simulink model "harmonic_comensation_simulation"  (R2020a)
settings: Solver=VariableStepAuto  StartTime=0.0  StopTime=3  RelTol=1e-3
values from neighbouring files (symbols this model uses):
  comp_table1 = [0.0466534535288 0.0494662824403 0.051313759182 0.0523377273586 0.0526570501043 0.0523721273536 0.0515686346954 0.0503206665416 0.0486934290661 0.0467455980054 0.0445314294364 0.0421026843564 ... (285300 elements, 951x300)]    [tables_50to1000.mat]
undefined symbols (not defined in the file or in its folder): B13, Bm, deltaT, DiscIntNeverNeededParam, J, Kd0, lam_pm, Ld, Lq, max_predq, P, Rs, run_comp, ss_d, ss_q, start_comp
libraries: simulink x1
settings Model: Creator=adamh  LastModifiedBy=adamh

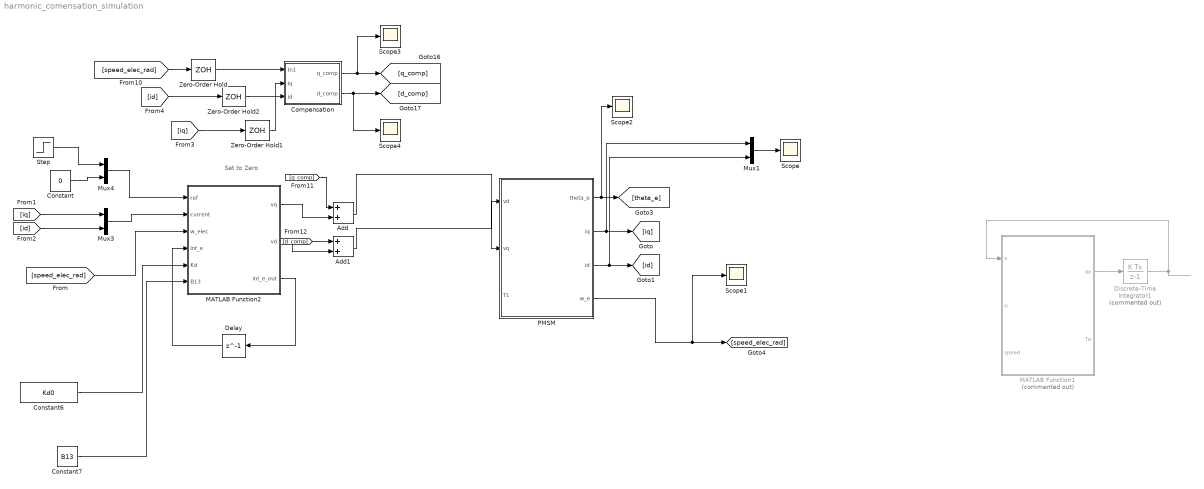
== system harmonic_comensation_simulation ==
  note: Set to Zero
  Add : Sum
  Add1 : Sum
  Compensation : Subsystem
  Constant : Constant  Value=0
  Constant6 : Constant  Value=Kd0
  Constant7 : Constant  Value=B13
  Delay : Delay  DelayLength=1  InitialCondition=[0.0; 0.0]
  Discrete-Time Integrator1 : DiscreteIntegrator  Commented=on  SampleTime=deltaT/100  ICPrevOutput=DiscIntNeverNeededParam  ICPrevScaledInput=DiscIntNeverNeededParam
  MATLAB Function1 : MATLAB Function  Commented=on  TreatAsAtomicUnit=on  SystemSampleTime=deltaT/100
  MATLAB Function2 : MATLAB Function  TreatAsAtomicUnit=on  SystemSampleTime=deltaT
  Mux1 : Mux  Inputs=2
  Mux3 : Mux  Inputs=2
  Mux4 : Mux  Inputs=2
  PMSM : Subsystem
  Scope{,1..4} (5 alike) : Scope
  Step : Step  Time=0  SampleTime=0
  Zero-Order Hold : ZeroOrderHold  SampleTime=deltaT
  Zero-Order Hold1 : ZeroOrderHold  SampleTime=deltaT
  Zero-Order Hold2 : ZeroOrderHold  SampleTime=deltaT
  wires:
  Constant6/1 -> MATLAB Function2/5(Kd)
  [d_comp] -> Add1/1
  Constant7/1 -> MATLAB Function2/6(B13)
  [q_comp] -> Add/1
  MATLAB Function2/2(vd) -> Add1/2
  Mux4/1 -> MATLAB Function2/1(ref)
  MATLAB Function2/1(vq) -> Add/2
  Delay/1 -> MATLAB Function2/4(int_e)
  Mux3/1 -> MATLAB Function2/2(current)
  [speed_elec_rad] -> MATLAB Function2/3(w_elec)
  Constant/1 -> Mux4/2
  [iq] -> Mux3/1
  [id] -> Mux3/2
  MATLAB Function2/3(int_e_out) -> Delay/1
  [speed_elec_rad] -> Zero-Order Hold/1
  Compensation/1(q_comp) -> Scope3/1, [q_comp]
  Compensation/2(d_comp) -> Scope4/1, [d_comp]
  Step/1 -> Mux4/1
  Zero-Order Hold/1 -> Compensation/1(In1)
  ? -> MATLAB Function1/2(u)
  Discrete-Time Integrator1/1 -> MATLAB Function1/1(x)
  MATLAB Function1/1(dx) -> Discrete-Time Integrator1/1
  Add/1 -> PMSM/2(vq)
  Add1/1 -> PMSM/1(vd)
  PMSM/4(w_e) -> Scope1/1, [speed_elec_rad]
  PMSM/1(theta_e) -> Scope2/1, [theta_e]
  PMSM/3(id) -> Mux1/2, [id]
  PMSM/2(iq) -> Mux1/1, [iq]
  Mux1/1 -> Scope/1
  [iq] -> Zero-Order Hold1/1
  [id] -> Zero-Order Hold2/1
  Zero-Order Hold1/1 -> Compensation/2(iq)
  Zero-Order Hold2/1 -> Compensation/3(id)

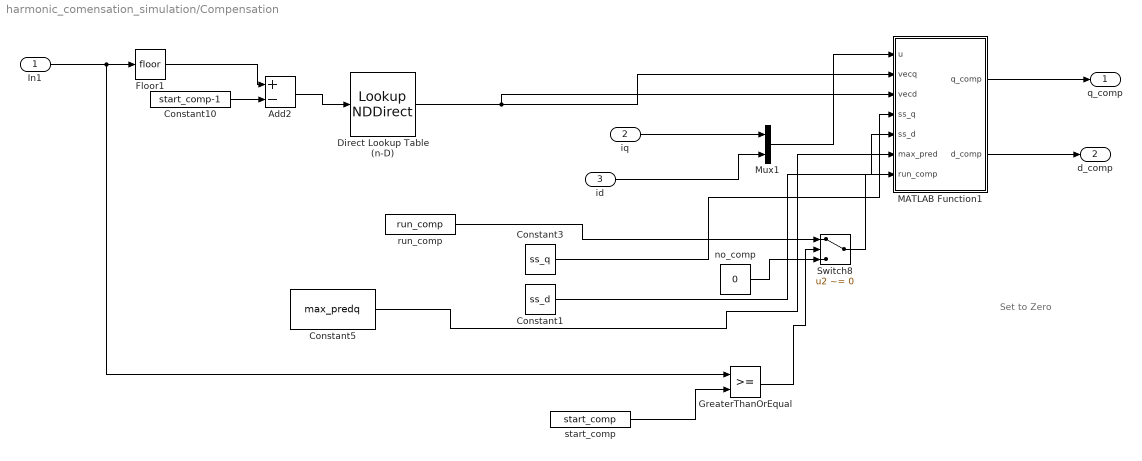
== system harmonic_comensation_simulation/Compensation ==
  note: Set to Zero
  In1 : Inport
  iq : Inport  Port=2
  id : Inport  Port=3
  Add2 : Sum  Inputs=+-
  Constant1 : Constant  Value=ss_d
  Constant10 : Constant  Value=start_comp-1
  Constant3 : Constant  Value=ss_q
  Constant5 : Constant  Value=max_predq
  Direct Lookup Table (n-D) : LookupNDDirect  InputsSelectThisObjectFromTable=Vector  Table=comp_table1'
  Floor1 : Rounding
  GreaterThanOrEqual : RelationalOperator  OutDataTypeStr=boolean  RndMeth=Simplest
  MATLAB Function1 : MATLAB Function  TreatAsAtomicUnit=on
  Mux1 : Mux  Inputs=2
  Switch8 : Switch  Criteria=u2 ~= 0
  no_comp : Constant  Value=0
  run_comp : Constant  Value=run_comp
  start_comp : Constant  Value=start_comp
  q_comp : Outport
  d_comp : Outport  Port=2
  wires:
  Add2/1 -> Direct Lookup Table (n-D)/1
  Direct Lookup Table (n-D)/1 -> MATLAB Function1/3(vecd), MATLAB Function1/2(vecq)
  GreaterThanOrEqual/1 -> Switch8/2
  id/1 -> Mux1/2
  run_comp/1 -> Switch8/1
  Mux1/1 -> MATLAB Function1/1(u)
  Constant10/1 -> Add2/2
  Floor1/1 -> Add2/1
  start_comp/1 -> GreaterThanOrEqual/2
  Constant5/1 -> MATLAB Function1/6(max_pred)
  Constant3/1 -> MATLAB Function1/4(ss_q)
  Constant1/1 -> MATLAB Function1/5(ss_d)
  no_comp/1 -> Switch8/3
  MATLAB Function1/2(d_comp) -> d_comp/1
  Switch8/1 -> MATLAB Function1/7(run_comp)
  MATLAB Function1/1(q_comp) -> q_comp/1
  In1/1 -> GreaterThanOrEqual/1, Floor1/1
  iq/1 -> Mux1/1

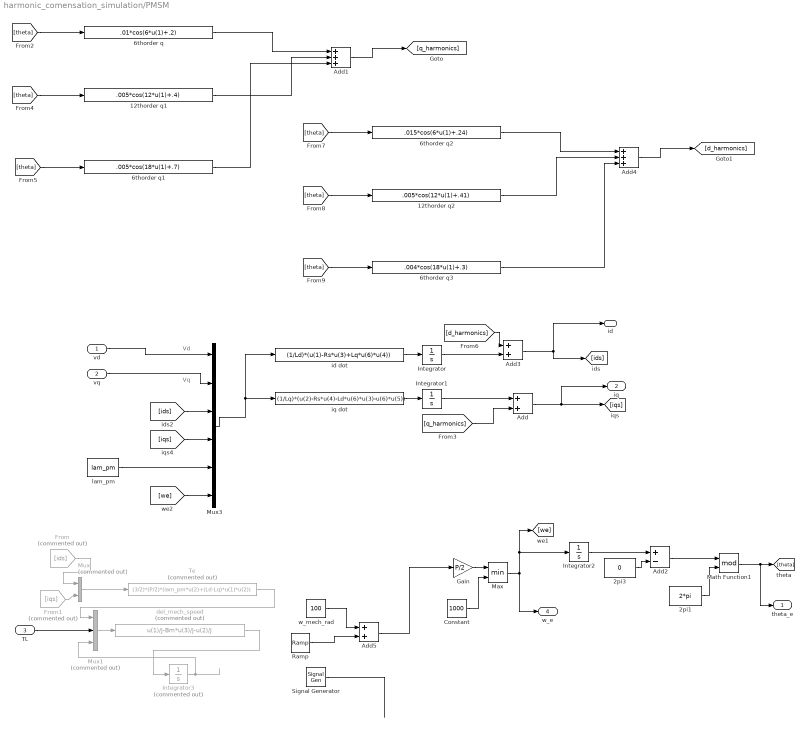
== system harmonic_comensation_simulation/PMSM ==
  note: Vq
  note: Vd
  vd : Inport
  vq : Inport  Port=2
  TL : Inport  Port=3
  12thorder q1 : Fcn  Expr=.005*cos(12*u(1)+.4)
  12thorder q2 : Fcn  Expr=.005*cos(12*u(1)+.41)
  2pi1 : Constant  Value=2*pi
  2pi3 : Constant  Value=0
  6thorder q : Fcn  Expr=.01*cos(6*u(1)+.2)
  6thorder q1 : Fcn  Expr=.005*cos(18*u(1)+.7)
  6thorder q2 : Fcn  Expr=.015*cos(6*u(1)+.24)
  6thorder q3 : Fcn  Expr=.004*cos(18*u(1)+.3)
  Add : Sum
  Add1 : Sum  Inputs=+++
  Add2 : Sum  Inputs=+-
  Add3 : Sum
  Add4 : Sum  Inputs=+++
  Add5 : Sum
  Constant : Constant  Value=1000
  From : From  Commented=on  GotoTag=ids
  From1 : From  Commented=on  GotoTag=iqs
  Gain : Gain  Gain=P/2
  Integrator : Integrator
  Integrator1 : Integrator
  Integrator2 : Integrator
  Integrator3 : Integrator  Commented=on
  Math Function1 : Math  Operator=mod  SignedPower=on  SaturateOnIntegerOverflow=on
  Max : MinMax  Inputs=2
  Mux : Mux  Commented=on  Inputs=2
  Mux1 : Mux  Commented=on  Inputs=3
  Mux3 : Mux  Inputs=6
  Ramp : simulink/Sources/Ramp  slope=25  start=1  InitialOutput=0
  Signal Generator : SignalGenerator  Amplitude=10  Units=rad/sec
  Te : Fcn  Commented=on  Expr=(3/2)*(P/2)*(lam_pm*u(2)+(Ld-Lq)*u(1)*u(2))
  del_mech_speed : Fcn  Commented=on  Expr=u(1)/J-Bm*u(3)/J-u(2)/J
  id dot : Fcn  Expr=(1/Ld)*(u(1)-Rs*u(3)+Lq*u(6)*u(4))
  iq dot : Fcn  Expr=(1/Lq)*(u(2)-Rs*u(4)-Ld*u(6)*u(3)-u(6)*u(5))
  lam_pm : Constant  Value=lam_pm
  w_mech_rad : Constant  Value=100
  theta_e : Outport  VectorParamsAs1DForOutWhenUnconnected=off
  iq : Outport  Port=2
  id : Outport  Port=3
  w_e : Outport  Port=4
  wires:
  Integrator/1 -> Add3/2
  iq dot/1 -> Integrator1/1
  id dot/1 -> Integrator/1
  vd/1 -> Mux3/1
  [iqs] -> Mux3/4
  Integrator2/1 -> Add2/1
  Mux3/1 -> iq dot/1, id dot/1
  [ids] -> Mux3/3
  lam_pm/1 -> Mux3/5
  [we] -> Mux3/6
  2pi1/1 -> Math Function1/2
  Math Function1/1 -> theta_e/1, [theta]
  2pi3/1 -> Add2/2
  Add2/1 -> Math Function1/1
  Integrator1/1 -> Add/1
  vq/1 -> Mux3/2
  Mux/1 -> Te/1
  From/1 -> Mux/1
  From1/1 -> Mux/2
  del_mech_speed/1 -> Integrator3/1
  Integrator3/1 -> Mux1/3
  Mux1/1 -> del_mech_speed/1
  Te/1 -> Mux1/1
  TL/1 -> Mux1/2
  6thorder q/1 -> Add1/1
  Add/1 -> iq/1, [iqs]
  [q_harmonics] -> Add/2
  12thorder q1/1 -> Add1/2
  6thorder q1/1 -> Add1/3
  Add1/1 -> [q_harmonics]
  [d_harmonics] -> Add3/1
  Add3/1 -> id/1, [ids]
  6thorder q3/1 -> Add4/3
  12thorder q2/1 -> Add4/2
  6thorder q2/1 -> Add4/1
  Add4/1 -> [d_harmonics]
  w_mech_rad/1 -> Add5/1
  Ramp/1 -> Add5/2
  Add5/1 -> Gain/1
  Gain/1 -> Max/1
  Constant/1 -> Max/2
  Max/1 -> Integrator2/1, [we], w_e/1
  Signal Generator/1 -> ?
  [theta] -> 6thorder q/1
  [theta] -> 6thorder q1/1
  [theta] -> 12thorder q1/1
  [theta] -> 6thorder q2/1
  [theta] -> 12thorder q2/1
  [theta] -> 6thorder q3/1

== matlab function harmonic_comensation_simulation/Compensation/MATLAB Function1 ==
  settings: updateMethod=DISCRETE
  data: u input; q_comp output; vecq input; vecd input; ss_q input; ss_d input; max_pred input; run_comp input; d_comp output
function [q_comp, d_comp]  = fcn(u,vecq,vecd, ss_q,ss_d, max_pred, run_comp)

    persistent delayq
    persistent q_pred
    persistent delayd
    persistent d_pred
    
    if isempty(delayq)  
        nEq = length(vecq);
        delayq = zeros(nEq,1);
    end
    if isempty(q_pred)  
        q_pred = 0;
    end
     if isempty(delayd)  
        nEd = length(vecd);
        delayd = zeros(nEd,1);
    end
    if isempty(d_pred)  
        d_pred = 0;
    end  

    
    % compensation
    %protection
    if abs(q_pred)>max_pred || run_comp == 0         
       delayq = [u(1);delayq(1:end-1)]; 
       q_pred = dot(vecq,delayq);
       q_comp=0;
    else

        delayq = [u(1)+q_pred;delayq(1:end-1)];
        q_pred = dot(vecq,delayq); % extract 
        q_comp = ss_q*q_pred;  
    end
    
    if abs(d_pred)>max_pred || run_comp == 0         
       delayd = [u(2);delayd(1:end-1)]; 
       d_pred = dot(vecd,delayd);
       d_comp=0;
    else
        delayd = [u(2)+d_pred;delayd(1:end-1)];
        d_pred = dot(vecd,delayd); % extract 
        d_comp = ss_d*d_pred; 
    end

== matlab function harmonic_comensation_simulation/MATLAB Function2 ==
  data: ref input size=2; current input size=2; w_elec input; int_e input size=2; vq output; vd output; int_e_out output; Kd input; B13 input
function [vq, vd, int_e_out] = traditional_LQI(ref,current,w_elec,int_e, Kd, B13)

% VDC = 42;

% from Real Parameters
% Ke =[1.6894   -0.1842    0.0000    0.3627   -1.7799    0.3569;
%     0.1842    1.6894   -0.3627    0.0000   -0.3569   -1.7799] ; 
% from fbedmdc
% Ke =[ 2.3940   -0.1699   -0.0016    0.5049   -2.5070    0.2027;
%     0.0938    2.4391   -0.5046   -0.0009   -0.1301   -2.5545];



e = ref - current;
int_e = int_e + e;
% int_e = int_e +Tsd2*e + Tsd2*old_e_in
Kd(1,2) = Kd(1,2)*w_elec;
% Ke(1,4) = Ke(1,4)*w_elec;
Kd(2,1) = Kd(2,1)*w_elec;
% Ke(2,3) = Ke(2,3)*w_elec;

% states = [u(1);u(2);u(1)*factor; u(2)*factor; int_e(1); int_e(2)];
states = [current(1);current(2); int_e(1); int_e(2)];

y = -Kd*states;
% y(1) = y(1) - B13*w_elec; % is B13 negative, should be
vq =y(1);
vd =y(2);

% vq = vq/VDC;
% vd =vd/VDC;

% vq = 0;
% vd = 0;


int_e_out = int_e;
% old_e = e;
% prevent integrator windup
% if vq ~= y(1) || vd ~= y(2)
%     %satureted
%     int_e_out = int_e - e;
% else
%     int_e_out = int_e;
% end

== matlab function harmonic_comensation_simulation/MATLAB Function1 ==
  data: x input size=4; u input size=2; dx output size=4; speed input; Te output; params parameter
function [dx, Te] = extended_pmsm_motor(x,u,speed, params)
    % extended dq model from Advanced Theory of Fractional-Slot
    % Concentrated Permanent Magnet Machines Thesis    

    % initial condition x(6) = .1631 Lq_dc    
    % initial condition x(7) = .1447 Ld_dc 
    % initial condition x(9) = .4055 Lamdapm_d
    
%     persistent dx_1_old dx_2_old  
%     if isempty(dx_1_old)
%         dx_1_old = 0;
%         dx_2_old = 0;
%     end
    
    vq = u(1);
    vd = u(2);

    rs = params.rs;
    Ld_dc = params.Ld_dc;
    Lq_dc = params.Lq_dc;
    lmda_f_dc = params.lmda_f_dc;
    P = params.Poles;    
    J = params.J;
    Bm = params.Bm;
    TL = params.TL;
    
    dx = zeros(4,1);   
    w = x(3);
    if params.spd_ctl  
        w = speed; 
    else
        w =x(3);
    end 
    
%     Mqd = 4.3600e-04*sin(6*x(4)*P/2);
%     d_Mqddt = .002616*cos(6*x(4)*P/2)*w*P/2;% derivative of mutual insuctance Mqddt
%     Lq_h = 6.6500e-04*cos(6*x(4)*P/2); % dc not included 0.1631
%     d_Lqdt =  -0.00399*sin(6.0*x(4)*P/2)*w*P/2; % derivative of Lq
%     Ld_h =   -3.5500e-04*cos(6*x(4)*P/2) ; % dc not included 0.1447 
%     d_Lddt = 0.00213*sin(6.0*x(4)*P/2)*w*P/2; % derivative of Ld
%     lmda_pm_q_h= 3.7000e-04*sin(6*x(4)*P/2);
%     d_lamqdt = 0.00222*cos(6.0*x(4)*P/2*P/2)*w*P/2; % derivative of lamda_pm_q
%     lmda_pm_d_h = 2.7000e-04*cos(6*x(4)*P/2);
%     d_lamddt = -0.00162*sin(6.0*x(4)*P/2)*w*P/2; % derivative of lamda_pm_d
    
    Mqd = 4.3600e-02*sin(6*x(4)*P/2);
    d_Mqddt = .2616*cos(6*x(4)*P/2)*w*P/2;% derivative of mutual insuctance Mqddt
    Lq_h = 6.6500e-02*cos(6*x(4)*P/2); % dc not included 0.1631
    d_Lqdt =  -0.399*sin(6.0*x(4)*P/2)*w*P/2; % derivative of Lq
    Ld_h =   -3.5500e-02*cos(6*x(4)*P/2) ; % dc not included 0.1447 
    d_Lddt = 0.213*sin(6.0*x(4)*P/2)*w*P/2; % derivative of Ld
    lmda_pm_q_h= 3.7000e-02*sin(6*x(4)*P/2);
    d_lamqdt = 0.222*cos(6.0*x(4)*P/2*P/2)*w*P/2; % derivative of lamda_pm_q
    lmda_pm_d_h = 2.7000e-02*cos(6*x(4)*P/2);
    d_lamddt = -0.162*sin(6.0*x(4)*P/2)*w*P/2; % derivative of lamda_pm_d    
    



    %vLq q axis voltage generated due to dependency of Lq Mqd and Mq0 on angle
    vLq = d_Lqdt*x(1)+d_Mqddt*x(2);
    vLd = d_Lddt*x(2)+d_Mqddt*x(1);
    %vlamq q-axis voltage generated due to the dependency of the q-axis
    %flux on angle
    vlamq = d_lamqdt;
    vlamd = d_lamddt;
%     viq q-axis voltage generated due to d-axis being function of time
%     viq = x(5)*dx_2_old; 
%     vid = x(5)*dx_1_old;
%     viq = Mqd*dx_2_old; 
% 
%     vid = Mqd*dx_1_old;    

    Lq_theta = Lq_dc + Lq_h;
    Ld_theta = Ld_dc + Ld_h;   
    lmda_q = Lq_theta*x(1);
%     lmda_pm_q = x(8);
%     lmda_pm_d = lmda_f_dc + x(9);
    lmda_pm_d = lmda_f_dc + lmda_pm_d_h;
    lmda_d = Ld_theta*x(2) + lmda_pm_d;

    
%     dx(1) = (1./Lq_theta).*(vq -rs*x(1) - lmda_d*P/2*w -vLq-vlamq-viq);% iq   
%     dx(2) = (1./Ld_theta).*(vd -rs*x(2) + lmda_q*P/2*w -vLd-vlamd-vid);% id 
    dx(1) = (1./Lq_theta).*(vq -rs*x(1) - lmda_d*P/2*w -vLq-vlamq);% iq   
    dx(2) = (1./Ld_theta).*(vd -rs*x(2) + lmda_q*P/2*w -vLd-vlamd);% id %    
%     dx_2_old = dx(2);
%     dx_1_old = dx(1);
    
    % Te = Tave+Trel+Tlam
    T_ave = (3/2)*(P/2)*(lmda_f_dc*x(1)+(Ld_dc-Lq_dc)*x(1)*x(2));
    % torque ripple T_rel and T_lam where T_lam dominates
    T_rel = 0; % not included yet
    % torque ripple from flux linkage harmonics
%     T_lam = -(3/2)*(P/2)*(x(1)*(x(9)-6*x(8)) + x(2)*(x(8)-6*x(9)));
    T_lam = -(3/2)*(P/2)*(x(1)*(lmda_pm_d_h-6*lmda_pm_q_h)...
        + x(2)*(lmda_pm_q_h-6*lmda_pm_d_h));
    Te = T_ave + T_rel + T_lam;
%     Te = T_ave;
    if params.spd_ctl  
        dx(3) = 0; % constant speed
    else
        dx(3) = Te/J-Bm*x(3)/J-TL/J;% mech speed
    end 
    
%     dx(4) = x(3);% mech angle
    

    
%     % second derivatives
%     dx(10) = -0.015696*(P/2*w)^2*sin(6.0*x(4)*P/2);% Mqd 2nd derivative
%     dx(11) =  -0.02394*(P/2*w)^2*cos(6.0*x(4)*P/2); % Lq 2nd derivative
%     dx(12) = 0.01278*(P/2*w)^2*cos(6.0*x(4)*P/2); % Ld 2nd derivative
%     dx(13) = -0.01332*(P/2*w)^2*sin(6.0*x(4)*P/2); % lamda_pm_q 2nd derivative
%     dx(14) = 0.00972*(P/2*w)^2*cos(6.0*x(4)*P/2); % lamda_pm_d 2nd derivative     
    
end
